simulink model "CP_SFC_NLin_n9945008"  (R2018b)
settings: Solver=ode4  StartTime=0.0  StopTime=5  FixedStep=0.02  MinStep=0.002  RelTol=1e-3
values from neighbouring files (symbols this model uses):
  g = 9.81    [CP_SFC_Lin_a_MainFile_n9945008.m]    (also in CP_SFC_Lin_b_MainFile_n9945008.m)
  K_SF = Ka    [CP_SFC_Lin_a_MainFile_n9945008.m]    (also in CP_SFC_Lin_b_MainFile_n9945008.m = Kb)
  l = 0.2    [CP_SFC_Lin_a_MainFile_n9945008.m]    (also in CP_SFC_Lin_b_MainFile_n9945008.m)
  m = 0.15    [CP_SFC_Lin_a_MainFile_n9945008.m]    (also in CP_SFC_Lin_b_MainFile_n9945008.m)
  Mc = 0.4    [CP_SFC_Lin_a_MainFile_n9945008.m]    (also in CP_SFC_Lin_b_MainFile_n9945008.m)
  setPoint = 0    [CP_SFC_Lin_a_MainFile_n9945008.m]    (also in CP_SFC_Lin_b_MainFile_n9945008.m = 3.14159265359)
  x0 = [0.2 20*pi/180 0 0]'    [CP_SFC_Lin_a_MainFile_n9945008.m]    (also in CP_SFC_Lin_b_MainFile_n9945008.m = [0.4 200*pi/180 0 0]')
settings Model: Creator=Cody  LastModifiedBy=Cody

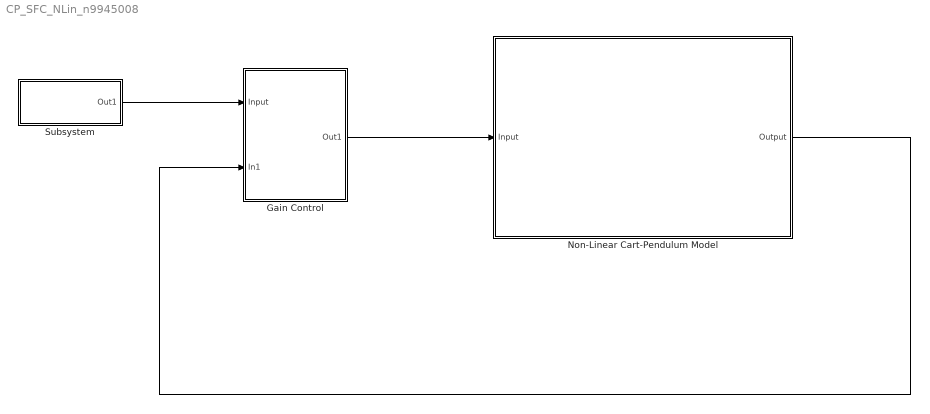
== system CP_SFC_NLin_n9945008 ==
  Gain Control : Subsystem
  "Non-Linear Cart-Pendulum Model " : Subsystem
  Subsystem : Subsystem
  wires:
  Gain Control/1(Out1) -> "Non-Linear Cart-Pendulum Model "/1(Input)
  "Non-Linear Cart-Pendulum Model "/1(Output) -> Gain Control/2(In1)
  Subsystem/1(Out1) -> Gain Control/1(Input)

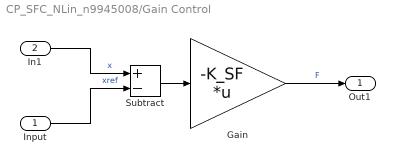
== system CP_SFC_NLin_n9945008/Gain Control ==
  Input : Inport
  In1 : Inport  Port=2
  Gain : Gain  Gain=-K_SF  Multiplication=Matrix(K*u)
  Subtract : Sum  Inputs=+-
  Out1 : Outport
  wires:
  Gain/1 -> Out1/1  "F"
  In1/1 -> Subtract/1  "x"
  Input/1 -> Subtract/2  "xref"
  Subtract/1 -> Gain/1

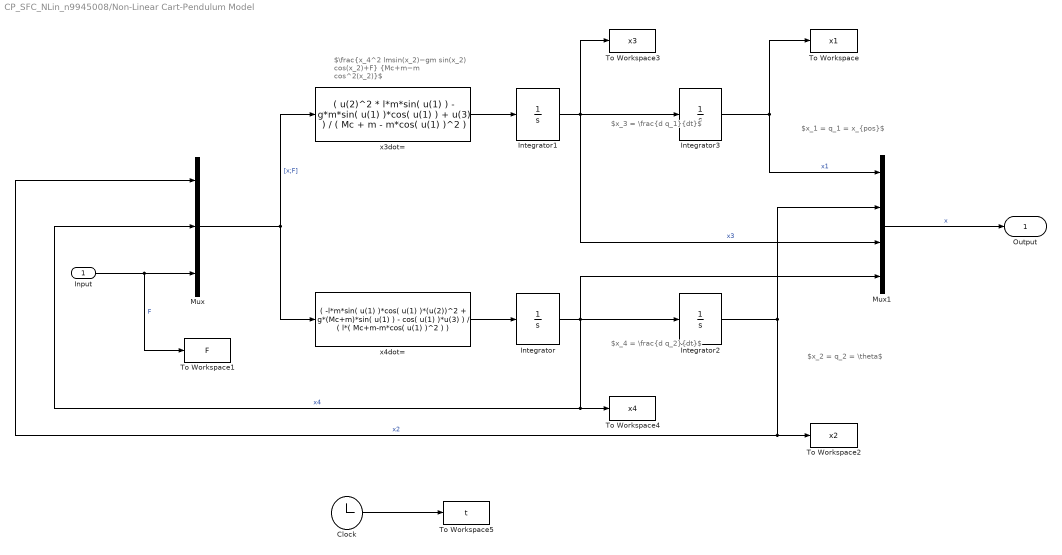
== system CP_SFC_NLin_n9945008/Non-Linear Cart-Pendulum Model  ==
  note: $\frac{x_4^2 lmsin(x_2)−gm sin(x_2) cos(x_2)+F} {Mc+m−m cos^2(x_2)}$
  note: $x_4 = \frac{d q_2}{dt}$
  note: $x_3 = \frac{d q_1}{dt}$
  note: $x_1 = q_1 = x_{pos}$
  note: $x_2 = q_2 = \theta$
  Input : Inport
  Clock : Clock
  Integrator : Integrator  InitialCondition=x0(4)
  Integrator1 : Integrator  InitialCondition=x0(3)
  Integrator2 : Integrator  InitialCondition=x0(2)  WrappedStateUpperValue=2*pi  WrappedStateLowerValue=0
  Integrator3 : Integrator  InitialCondition=x0(1)
  Mux : Mux  Inputs=3
  Mux1 : Mux
  To Workspace : ToWorkspace  VariableName=x1  SampleTime=-1
      settings: Save2DSignal=2-D array (concatenate along first dimension)
  To Workspace1 : ToWorkspace  VariableName=F  SampleTime=-1
      settings: Save2DSignal=2-D array (concatenate along first dimension)
  To Workspace2 : ToWorkspace  VariableName=x2  SampleTime=-1
      settings: Save2DSignal=2-D array (concatenate along first dimension)
  To Workspace3 : ToWorkspace  VariableName=x3  SampleTime=-1
      settings: Save2DSignal=2-D array (concatenate along first dimension)
  To Workspace4 : ToWorkspace  VariableName=x4  SampleTime=-1
      settings: Save2DSignal=2-D array (concatenate along first dimension)
  To Workspace5 : ToWorkspace  VariableName=t  SampleTime=-1
      settings: Save2DSignal=2-D array (concatenate along first dimension)
  "x3dot= " : Fcn  Expr="(  u(2)^2 * l*m*sin( u(1) ) - g*m*sin( u(1) )*cos( u(1) ) + u(3)  )  /  (  Mc + m - m*cos( u(1) )^2  )"
  "x4dot= " : Fcn  Expr="(  -l*m*sin( u(1) )*cos( u(1) )*(u(2))^2 + g*(Mc+m)*sin( u(1) ) - cos( u(1) )*u(3)  )  /  (  l*( Mc+m-m*cos( u(1) )^2 )  )"
  Output : Outport
  wires:
  Integrator/1 -> Mux/2, To Workspace4/1, Mux1/4, Integrator2/1  "x4"
  Clock/1 -> To Workspace5/1
  Input/1 -> Mux/3, To Workspace1/1  "F"
  Integrator1/1 -> Mux1/3, Integrator3/1, To Workspace3/1  "x3"
  "x3dot= "/1 -> Integrator1/1
  Mux/1 -> "x4dot= "/1, "x3dot= "/1  "[x;F]"
  "x4dot= "/1 -> Integrator/1
  Integrator3/1 -> Mux1/1, To Workspace/1  "x1"
  Integrator2/1 -> Mux/1, To Workspace2/1, Mux1/2  "x2"
  Mux1/1 -> Output/1  "x"

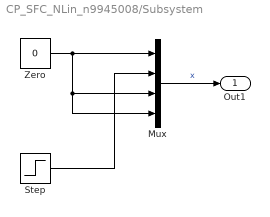
== system CP_SFC_NLin_n9945008/Subsystem ==
  Mux : Mux
  Step : Step  Time=0  After=setPoint  SampleTime=0
  Zero : Constant  Value=0  OutDataTypeStr=Inherit: Inherit via back propagation
  Out1 : Outport
  wires:
  Mux/1 -> Out1/1  "x"
  Zero/1 -> Mux/4, Mux/3, Mux/1
  Step/1 -> Mux/2
